simulink library "performanceIndexComponents"  (R2017b)
settings: Solver=VariableStepAuto  StartTime=0.0  StopTime=10.0  RelTol=1e-3
undefined symbols (not defined in the file): p
settings Model: Creator=M.Cobb  LastModifiedBy=mitch

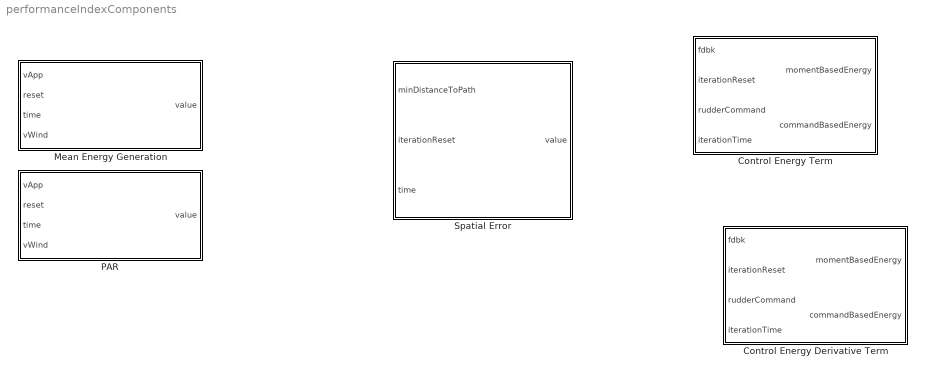
== system performanceIndexComponents ==
  Control Energy Derivative Term : Subsystem
  Control Energy Term : Subsystem
  Mean Energy Generation : Subsystem
  PAR : Subsystem
  Spatial Error : Subsystem

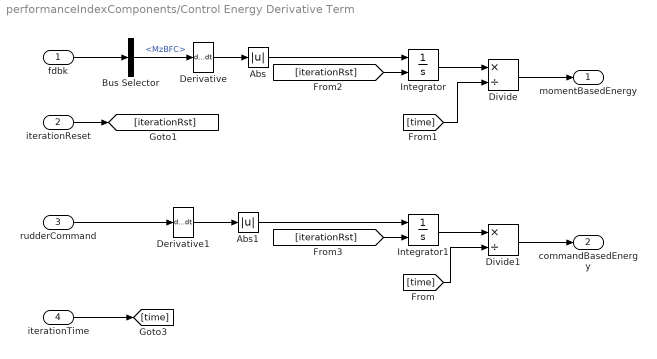
== system performanceIndexComponents/Control Energy Derivative Term ==
  fdbk : Inport
  iterationReset : Inport  Port=2
  rudderCommand : Inport  Port=3
  iterationTime : Inport  Port=4
  Abs : Abs
  Abs1 : Abs
  Bus Selector : BusSelector  OutputSignals=MzBFC
  Derivative : Derivative
  Derivative1 : Derivative
  Divide : Product  Inputs=*/
  Divide1 : Product  Inputs=*/
  Integrator : Integrator  ExternalReset=rising
  Integrator1 : Integrator  ExternalReset=rising
  momentBasedEnergy : Outport
  commandBasedEnergy : Outport  Port=2
  wires:
  Bus Selector/1 -> Derivative/1  "<MzBFC>"
  fdbk/1 -> Bus Selector/1
  Abs/1 -> Integrator/1
  rudderCommand/1 -> Derivative1/1
  Abs1/1 -> Integrator1/1
  iterationTime/1 -> [time]
  Integrator/1 -> Divide/1
  Divide/1 -> momentBasedEnergy/1
  Divide1/1 -> commandBasedEnergy/1
  Integrator1/1 -> Divide1/1
  [time] -> Divide1/2
  [time] -> Divide/2
  iterationReset/1 -> [iterationRst]
  [iterationRst] -> Integrator/2
  [iterationRst] -> Integrator1/2
  Derivative/1 -> Abs/1
  Derivative1/1 -> Abs1/1

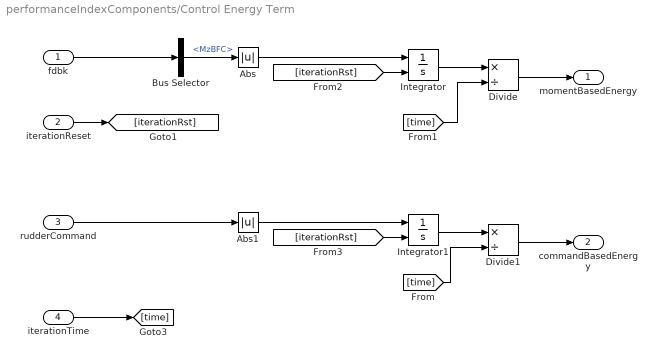
== system performanceIndexComponents/Control Energy Term ==
  fdbk : Inport
  iterationReset : Inport  Port=2
  rudderCommand : Inport  Port=3
  iterationTime : Inport  Port=4
  Abs : Abs
  Abs1 : Abs
  Bus Selector : BusSelector  OutputSignals=MzBFC
  Divide : Product  Inputs=*/
  Divide1 : Product  Inputs=*/
  Integrator : Integrator  ExternalReset=rising
  Integrator1 : Integrator  ExternalReset=rising
  momentBasedEnergy : Outport
  commandBasedEnergy : Outport  Port=2
  wires:
  Bus Selector/1 -> Abs/1  "<MzBFC>"
  fdbk/1 -> Bus Selector/1
  Abs/1 -> Integrator/1
  rudderCommand/1 -> Abs1/1
  Abs1/1 -> Integrator1/1
  iterationTime/1 -> [time]
  Integrator/1 -> Divide/1
  Divide/1 -> momentBasedEnergy/1
  Divide1/1 -> commandBasedEnergy/1
  Integrator1/1 -> Divide1/1
  [time] -> Divide1/2
  [time] -> Divide/2
  iterationReset/1 -> [iterationRst]
  [iterationRst] -> Integrator/2
  [iterationRst] -> Integrator1/2

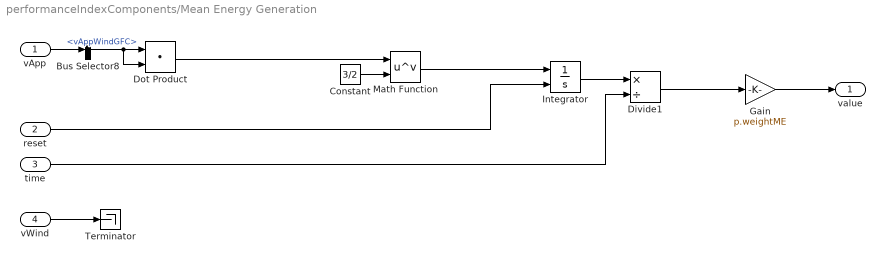
== system performanceIndexComponents/Mean Energy Generation ==
  vApp : Inport
  reset : Inport  Port=2
  time : Inport  Port=3
  vWind : Inport  Port=4
  Bus Selector8 : BusSelector  OutputSignals=vAppWindGFC
  Constant : Constant  Value=3/2
  Divide1 : Product  Inputs=*/
  Dot Product : DotProduct  InputSameDT=on  OutDataTypeStr=Inherit: Inherit via internal rule
  Gain : Gain  Gain=p.weightME
  Integrator : Integrator  ExternalReset=rising
  Math Function : Math  Operator=pow  SaturateOnIntegerOverflow=on
  Terminator : Terminator
  value : Outport
  wires:
  time/1 -> Divide1/2
  reset/1 -> Integrator/2
  Integrator/1 -> Divide1/1
  Constant/1 -> Math Function/2
  Math Function/1 -> Integrator/1
  Dot Product/1 -> Math Function/1
  vApp/1 -> Bus Selector8/1
  Bus Selector8/1 -> Dot Product/2, Dot Product/1  "<vAppWindGFC>"
  vWind/1 -> Terminator/1
  Divide1/1 -> Gain/1
  Gain/1 -> value/1

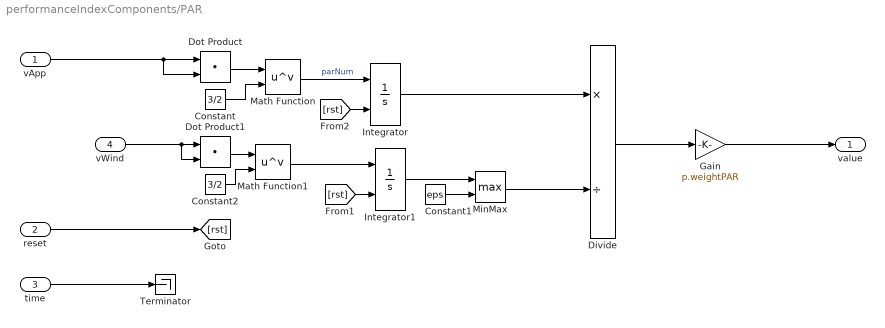
== system performanceIndexComponents/PAR ==
  vApp : Inport
  reset : Inport  Port=2
  time : Inport  Port=3
  vWind : Inport  Port=4
  Constant : Constant  Value=3/2
  Constant1 : Constant  Value=eps
  Constant2 : Constant  Value=3/2
  Divide : Product  Inputs=*/
  Dot Product : DotProduct  InputSameDT=on  OutDataTypeStr=Inherit: Inherit via internal rule
  Dot Product1 : DotProduct  InputSameDT=on  OutDataTypeStr=Inherit: Inherit via internal rule
  Gain : Gain  Gain=p.weightPAR
  Integrator : Integrator  ExternalReset=rising
  Integrator1 : Integrator  ExternalReset=rising
  Math Function : Math  Operator=pow  SaturateOnIntegerOverflow=on
  Math Function1 : Math  Operator=pow  SaturateOnIntegerOverflow=on
  MinMax : MinMax  Function=max  Inputs=2
  Terminator : Terminator
  value : Outport
  wires:
  vWind/1 -> Dot Product1/2, Dot Product1/1
  reset/1 -> [rst]
  Dot Product/1 -> Math Function/1
  Dot Product1/1 -> Math Function1/1
  MinMax/1 -> Divide/2
  Constant1/1 -> MinMax/2
  Constant/1 -> Math Function/2
  Constant2/1 -> Math Function1/2
  [rst] -> Integrator/2
  Math Function/1 -> Integrator/1  "parNum"
  Integrator/1 -> Divide/1
  [rst] -> Integrator1/2
  Math Function1/1 -> Integrator1/1
  Integrator1/1 -> MinMax/1
  vApp/1 -> Dot Product/2, Dot Product/1
  time/1 -> Terminator/1
  Divide/1 -> Gain/1
  Gain/1 -> value/1

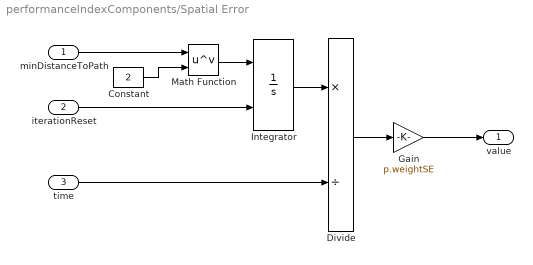
== system performanceIndexComponents/Spatial Error ==
  minDistanceToPath : Inport
  iterationReset : Inport  Port=2
  time : Inport  Port=3
  Constant : Constant  Value=2
  Divide : Product  Inputs=*/
  Gain : Gain  Gain=p.weightSE
  Integrator : Integrator  ExternalReset=rising
  Math Function : Math  Operator=pow  SaturateOnIntegerOverflow=on
  value : Outport
  wires:
  Math Function/1 -> Integrator/1
  minDistanceToPath/1 -> Math Function/1
  iterationReset/1 -> Integrator/2
  Constant/1 -> Math Function/2
  Integrator/1 -> Divide/1
  time/1 -> Divide/2
  Divide/1 -> Gain/1
  Gain/1 -> value/1
